simulink model "temperature_control"  (R2021b)
settings: Solver=VariableStepAuto  StartTime=0.0  StopTime=10.0  RelTol=1e-3
libraries: simulink x1
settings Model: Creator=ASA  LastModifiedBy=sa

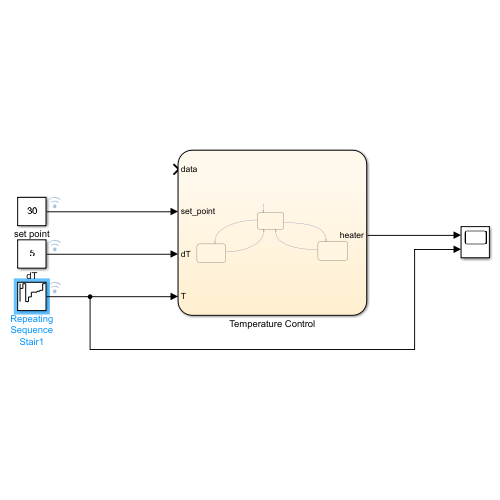
[thumbnail: Simulink's stored preview of the top-level diagram]
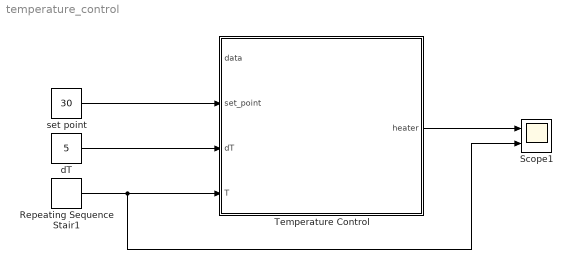
== system temperature_control ==
  Repeating Sequence Stair1 : simulink/Sources/Repeating Sequence Stair  OutValues=[40 50 10 20 30 31 32 35 50].'  tsamp=-1  OutMin=[]  OutMax=[]  OutDataTypeStr=double  OutputDataTypeScalingMode=double  OutDataType=fixdt(0,8)  ConRadixGroup=Best Precision: Vector-wise  OutScaling=2^-12
  Scope1 : Scope  NumInputPorts=2
  Temperature Control : Stateflow chart  TreatAsAtomicUnit=on
  dT : Constant  Value=5
  set point : Constant  Value=30
  wires:
  Repeating Sequence Stair1/1 -> Scope1/2, Temperature Control/4(T)
  set point/1 -> Temperature Control/2(set_point)
  dT/1 -> Temperature Control/3(dT)
  Temperature Control/1(heater) -> Scope1/1

== stateflow chart temperature_control/Temperature Control ==
  state off
    entry: heater = 0
  state Cool
    entry: heater = -1
  state Heat
    entry: heater = 1
  (default) -> off
  off -> Heat [order 1] : [T < (set_point - dT)]
  off -> Cool [order 2] : [T > (set_point + dT)]
  Heat -> off : [T >= (set_point - dT)]
  Cool -> off : [T <= (set_point + dT)]
  data: data input; set_point input; dT input; heater output; T input
